simulink model "Drone2_simulink_old1"  (R2024b)
settings: Solver=ode1be  StartTime=0.0  StopTime=1200  FixedStep=0.001  MaxStep=0.001  MinStep=0.00095  RelTol=1e-3
undefined symbols (not defined in the file): DiscIntNeverNeededParam, Environment, Newton, Raphson, Sim3dSensor, Vehicle, X, Y, Z
libraries: sm_lib x2951, nesl_utility x76, slpidlib x25, simulink x4, eeGeneralControl x4, matrix_library x3, rllib x2, sim3dlib x2, uavsim3dlib x2, dspstat3 x1, SignalEditorBlockLib x1, sharedutil x1
(part 10 of 21)

== system Drone2_simulink_old1/Drive Controls/Thrust Controls/Depth and Pitch Control/Main Propellers Thrust Offset Compensation ==
  PPf : Inport
  SPf : Inport  Port=2
  Bow Vertical Thruster Moment Arm : Constant  Value=-Vehicle.Thruster.BVarmX
  Main Propellers Moment Arm : Constant  Value=-Vehicle.Prop.SParmZ
  Product : Product
  Product1 : Product
  Product2 : Product  Inputs=*/
  Stern Vertical Thruster Moment Arm : Constant  Value=Vehicle.Thruster.SVarmX
  Sum : Sum  Inputs=|++
  Sum1 : Sum  Inputs=|++
  VTf : Outport
  wires:
  Product1/1 -> Sum/1
  Product/1 -> Sum/2
  SPf/1 -> Product/1
  PPf/1 -> Product1/1
  Main Propellers Moment Arm/1 -> Product1/2, Product/2
  Bow Vertical Thruster Moment Arm/1 -> Sum1/1
  Stern Vertical Thruster Moment Arm/1 -> Sum1/2
  Sum/1 -> Product2/1
  Sum1/1 -> Product2/2
  Product2/1 -> VTf/1

== system Drone2_simulink_old1/Drive Controls/Thrust Controls/Heading and Yaw Control/psidot ==
  pqr : Inport
  phithetapsi : Inport  Port=2
  Mux1 : Mux  Inputs=[3 3 3]
  psidot : Fcn  Expr=(u[2]*u[4]+u[3]*u[7])/u[8]
  sincos : Trigonometry  Operator=sincos
  psid : Outport  Unit=rad/s  InitialOutput=0  VectorParamsAs1DForOutWhenUnconnected=off
  wires:
  sincos/2 -> Mux1/3
  sincos/1 -> Mux1/2
  phithetapsi/1 -> sincos/1
  pqr/1 -> Mux1/1
  Mux1/1 -> psidot/1
  psidot/1 -> psid/1

== system Drone2_simulink_old1/Drive Controls/Thrust Controls/Heading and Yaw Control/side slip compensation ==
  note: NOTE: Lateral force offset is distributed based of the horizontal thrusters moment arms to make the net torque contribution zero
  v : Inport
  BowHTForce : Gain  Gain=Vehicle.Thruster.SHarmX/(-Vehicle.Thruster.BHarmX+Vehicle.Thruster.SHarmX)
  Gain1 : Gain  Gain=-1
  PIv : slpidlib/PID Controller  Controller=PI  Form=Parallel  TimeDomain=Continuous-time  UseExternalTs=off  SampleTime=-1  IntegratorMethod=Forward Euler  FilterMethod=Forward Euler  ControllerParametersSource=internal  P=10  I=0.01  UseKiTs=off  D=0  UseExternalDerivativeSource=off  N=100  UseFilter=on  TunerSelectOption=Transfer Function Based (PID Tuner App)  InitialConditionSource=internal  InitialConditionForIntegrator=0  InitialConditionForFilter=0  DifferentiatorICPrevScaledInput=0  ExternalReset=none  TrackingMode=off  Kt=1  LimitOutput=off  SatLimitsSource=internal  UpperSaturationLimit=inf  LowerSaturationLimit=-inf  LinearizeAsGain=on  AntiWindupMode=none  Kb=1  LimitIntegrator=off  UpperIntegratorSaturationLimit=inf  LowerIntegratorSaturationLimit=-inf  POutMin=[]  POutMax=[]  IOutMin=[]  IOutMax=[]  DOutMin=[]  DOutMax=[]  NOutMin=[]  NOutMax=[]  SumOutMin=[]  SumOutMax=[]  SaturationOutMin=[]  SaturationOutMax=[]  PParamMin=[]  PParamMax=[]  IParamMin=[]  IParamMax=[]  DParamMin=[]  DParamMax=[]  NParamMin=[]  NParamMax=[]  KbParamMin=[]  KbParamMax=[]  KtParamMin=[]  KtParamMax=[]  KbOutMin=[]  KbOutMax=[]  KtOutMin=[]  KtOutMax=[]  IntegratorOutMin=[]  IntegratorOutMax=[]  FilterOutMin=[]  FilterOutMax=[]  SumI1OutMin=[]  SumI1OutMax=[]  SumI2OutMin=[]  SumI2OutMax=[]  SumI3OutMin=[]  SumI3OutMax=[]  SumI4OutMin=[]  SumI4OutMax=[]  SumDOutMin=[]  SumDOutMax=[]  DifferentiatorOutMin=[]  DifferentiatorOutMax=[]  FilterDiffOutCoefMin=[]  FilterDiffOutCoefMax=[]  ReciprocalOutMin=[]  ReciprocalOutMax=[]  SumDenOutMin=[]  SumDenOutMax=[]  SumNumOutMin=[]  SumNumOutMax=[]  DivideOutMin=[]  DivideOutMax=[]  UdiffTsProdOutMin=[]  UdiffTsProdOutMax=[]  NTsProdOutMin=[]  NTsProdOutMax=[]  UintegralTsProdOutMin=[]  UintegralTsProdOutMax=[]  UngainTsProdOutMin=[]  UngainTsProdOutMax=[]  ClampingZeroOutDataTypeStr=Inherit: Inherit via back propagation  ClampingZeroOutMin=[]  ClampingZeroOutMax=[]  FilterDenConstantOutDataTypeStr=Inherit: Inherit via back propagation  FilterDenConstantOutMin=[]  FilterDenConstantOutMax=[]  PCopyOutDataTypeStr=Inherit: Inherit via back propagation  PCopyOutMin=[]  PCopyOutMax=[]  NCopyOutDataTypeStr=Inherit: Inherit via back propagation  NCopyOutMin=[]  NCopyOutMax=[]  IntegratorContinuousStateAttributes=''  IntegratorStateMustResolveToSignalObject=off  IntegratorRTWStateStorageClass=Auto  FilterContinuousStateAttributes=''  FilterStateMustResolveToSignalObject=off  FilterRTWStateStorageClass=Auto  ParallelPVariant=InternalParameters  IdealPVariant=Disabled  IVariant=InternalParameters  DVariant=Disabled  IntegratorVariant=Continuous  SatVariant=Disabled  AWVariant=Passthrough  PCopyVariant=Disabled  TRVariant=Disabled  FdbkBlocksVariant=Forward  IdealPFdbkVariant=Disabled  SatFdbkVariant=Disabled  DerivativeFilterVariant=Disabled  NVariant=Disabled  NCopyVariant=Disabled_SignalSpec  FilterICVariant=Disabled  IntegratorICVariant=InternalICs  ExternalResetVariant=Disabled  TRSumVariant=Passthrough  SumFdbkVariant=Disabled  SumVariant=Sum_PI  TsampFilterVariant=InternalTs  TsampNgainVariant=Passthrough  TsampIntegralVariant=Disabled_SignalSpec  ExternalSaturationOutDataTypeStr=Inherit: Same as second input  DerivativeSourceVariant=Disabled
  SternHTForce : Gain  Gain=-Vehicle.Thruster.BHarmX/(-Vehicle.Thruster.BHarmX+Vehicle.Thruster.SHarmX)
  BHTf : Outport
  SHTf : Outport  Port=2
  wires:
  Gain1/1 -> PIv/1
  SternHTForce/1 -> SHTf/1
  PIv/1 -> BowHTForce/1, SternHTForce/1
  v/1 -> Gain1/1
  BowHTForce/1 -> BHTf/1

== system Drone2_simulink_old1/Hydrostatic & Hydrodynamic Effects/Added Mass Forces/Added Mass/LPfilter ==
  note: NOTE:
      | Using low pass filters with
      | 1 milisecond time constant
      | to break the algebraic loop
  in : Inport
  Demux : Demux  Outputs=6
  LPfilter{1..6} (6 alike) : TransferFcn  Denominator=[0.001 1]
  Mux : Mux  Inputs=6
  out : Outport
  wires:
  Demux/1 -> LPfilter1/1
  Demux/2 -> LPfilter2/1
  in/1 -> Demux/1
  Demux/6 -> LPfilter6/1
  Demux/5 -> LPfilter5/1
  Demux/4 -> LPfilter4/1
  Demux/3 -> LPfilter3/1
  LPfilter1/1 -> Mux/1
  LPfilter2/1 -> Mux/2
  LPfilter3/1 -> Mux/3
  LPfilter4/1 -> Mux/4
  LPfilter5/1 -> Mux/5
  LPfilter6/1 -> Mux/6
  Mux/1 -> out/1

== system Drone2_simulink_old1/Hydrostatic & Hydrodynamic Effects/Added Mass Forces/Coriolis/Ca(V) ==
  note: $a_1 = m_{11}u \\ a_2 = m_{22}v+m_{26}r\\ a_3 = m_{33}w+m_{35}q\\ b_1 = m_{44}p\\ b_2 = m_{53}w+m_{55}q\\ b_3 = m_{62}v+m_{66}r$
  a1 : Inport
  a2 : Inport  Port=2
  a3 : Inport  Port=3
  b1 : Inport  Port=4
  b2 : Inport  Port=5
  b3 : Inport  Port=6
  Matrix Concatenate : Concatenate  NumInputs=6  Mode=Multidimensional array
  row1 : Subsystem
  row2 : Subsystem
  row3 : Subsystem
  row4 : Subsystem
  row5 : Subsystem
  row6 : Subsystem
  Ca(V) : Outport
  wires:
  a2/1 -> row1/1(a2), row3/2(a2), row6/2(a2), row4/1(a2)
  b3/1 -> row5/4(b3), row4/4(b3)
  b2/1 -> row4/3(b2), row6/4(b2)
  a1/1 -> row6/1(a1), row5/1(a1), row3/1(a1), row2/1(a1)
  row1/1(row1) -> Matrix Concatenate/1
  row2/1(row2) -> Matrix Concatenate/2
  row3/1(row3) -> Matrix Concatenate/3
  a3/1 -> row5/2(a3), row4/2(a3), row1/2(a3), row2/2(a3)
  row4/1(row4) -> Matrix Concatenate/4
  b1/1 -> row5/3(b1), row6/3(b1)
  row6/1(row6) -> Matrix Concatenate/6
  row5/1(row5) -> Matrix Concatenate/5
  Matrix Concatenate/1 -> Ca(V)/1

== system Drone2_simulink_old1/Hydrostatic & Hydrodynamic Effects/Drag Sub system/Aerodynamic drag/Area ==
  Area for rotation : Constant  Value=diag([C_x C_y C_z])  mask{C_x=Vehicle.Body.YZArea, C_y=Vehicle.Body.XZArea, C_z=Vehicle.Body.XYArea}
      mask prompts: C_x "Ax"; C_y "Ay"; C_z "Az"
      mask DialogControl DescGroupVar Prompt: Diagonal Matrix
      mask DialogControl DescTextVar Prompt: Provide values of diagonal element tp produce a diagonal matrix
      mask Display: disp('diag([Ax Ay Az])');
  Area for rotation1 : Constant  Value=diag([C_x C_y C_z])  mask{C_x=Vehicle.Body.Hulldiameter/2, C_y=Vehicle.Body.Length/2, C_z=Vehicle.Body.Length/2}
      mask prompts: C_x "Ax"; C_y "Ay"; C_z "Az"
      mask DialogControl DescGroupVar Prompt: Diagonal Matrix
      mask DialogControl DescTextVar Prompt: Provide values of diagonal element tp produce a diagonal matrix
      mask Display: disp('diag([Ax Ay Az])');
  Constant3 : Constant  Value=3
  Power : Math  Operator=pow
  Product2 : Product  Multiplication=Matrix(*)
  Linear : Outport
  Rotational : Outport  Port=2
  wires:
  Area for rotation1/1 -> Power/1
  Constant3/1 -> Power/2
  Area for rotation/1 -> Product2/1, Linear/1
  Power/1 -> Product2/2
  Product2/1 -> Rotational/1

== system Drone2_simulink_old1/Hydrostatic & Hydrodynamic Effects/Drag Sub system/Aerodynamic drag/Subsystem ==
  V_b : Inport
  rho : Inport  Port=2
  Abs : Abs  SaturateOnIntegerOverflow=off
  Product2 : Product
  Product3 : Product
  0.5rhov^2 : Outport
  wires:
  rho/1 -> Product3/2
  V_b/1 -> Abs/1, Product2/1
  Product3/1 -> 0.5rhov^2/1
  Abs/1 -> Product2/2
  Product2/1 -> Product3/1

== system Drone2_simulink_old1/Hydrostatic & Hydrodynamic Effects/Drag Sub system/Aerodynamic drag/Subsystem1 ==
  omega_b : Inport
  rho : Inport  Port=2
  Abs : Abs  SaturateOnIntegerOverflow=off
  Product2 : Product
  Product3 : Product
  0.5rhov^2 : Outport
  wires:
  Abs/1 -> Product2/2
  omega_b/1 -> Product2/1, Abs/1
  Product2/1 -> Product3/1
  rho/1 -> Product3/2
  Product3/1 -> 0.5rhov^2/1

== system Drone2_simulink_old1/Hydrostatic & Hydrodynamic Effects/Drag Sub system/Hydrodyanamic drag/Area ==
  Area for rotation : Constant  Value=diag([C_x C_y C_z])  mask{C_x=Vehicle.Body.YZArea, C_y=Vehicle.Body.XZArea, C_z=Vehicle.Body.XYArea}
      mask prompts: C_x "Ax"; C_y "Ay"; C_z "Az"
      mask DialogControl DescGroupVar Prompt: Diagonal Matrix
      mask DialogControl DescTextVar Prompt: Provide values of diagonal element tp produce a diagonal matrix
      mask Display: disp('diag([Ax Ay Az])');
  Area for rotation1 : Constant  Value=diag([C_x C_y C_z])  mask{C_x=Vehicle.Body.Hulldiameter/2, C_y=Vehicle.Body.Length/2, C_z=Vehicle.Body.Length/2}
      mask prompts: C_x "Ax"; C_y "Ay"; C_z "Az"
      mask DialogControl DescGroupVar Prompt: Diagonal Matrix
      mask DialogControl DescTextVar Prompt: Provide values of diagonal element tp produce a diagonal matrix
      mask Display: disp('diag([Ax Ay Az])');
  Constant3 : Constant  Value=3
  Power : Math  Operator=pow
  Product2 : Product  Multiplication=Matrix(*)
  Linear : Outport
  Rotational : Outport  Port=2
  wires:
  Product2/1 -> Rotational/1
  Area for rotation1/1 -> Power/1
  Constant3/1 -> Power/2
  Area for rotation/1 -> Product2/1, Linear/1
  Power/1 -> Product2/2

== system Drone2_simulink_old1/Hydrostatic & Hydrodynamic Effects/Drag Sub system/Hydrodyanamic drag/Subsystem ==
  V_b : Inport
  rho : Inport  Port=2
  Dot Product : DotProduct  OutDataTypeStr=Inherit: Inherit via internal rule
  Product2 : Product
  Product3 : Product
  Reshape : Reshape  OutputDimensionality=Customize  OutputDimensions=[3,1]
  Sqrt : Sqrt
  Transpose : Math  Operator=transpose
  0.5rhov^2 : Outport
  wires:
  V_b/1 -> Product2/1, Reshape/1, Transpose/1
  Sqrt/1 -> Product2/2
  Transpose/1 -> Dot Product/1
  Dot Product/1 -> Sqrt/1
  Product3/1 -> 0.5rhov^2/1
  Product2/1 -> Product3/1
  rho/1 -> Product3/2
  Reshape/1 -> Dot Product/2

== system Drone2_simulink_old1/Hydrostatic & Hydrodynamic Effects/Drag Sub system/Hydrodyanamic drag/Subsystem1 ==
  omega_b : Inport
  rho : Inport  Port=2
  Dot Product : DotProduct  OutDataTypeStr=Inherit: Inherit via internal rule
  Product2 : Product
  Product3 : Product
  Sqrt : Sqrt
  Transpose : Math  Operator=transpose
  0.5rhov^2 : Outport
  wires:
  rho/1 -> Product3/2
  omega_b/1 -> Transpose/1, Product2/1, Dot Product/1
  Product3/1 -> 0.5rhov^2/1
  Sqrt/1 -> Product2/2
  Product2/1 -> Product3/1
  Dot Product/1 -> Sqrt/1
  Transpose/1 -> Dot Product/2

== system Drone2_simulink_old1/Hydrostatic & Hydrodynamic Effects/Drag Sub system/Subsystem/Subsystem ==
  vector : Inport
  Dot Product : DotProduct  OutDataTypeStr=Inherit: Inherit via internal rule
  Reshape : Reshape  OutputDimensionality=Customize  OutputDimensions=[3,1]
  Sqrt : Sqrt
  Transpose : Math  Operator=transpose
  Magnitude : Outport
  wires:
  Sqrt/1 -> Magnitude/1
  Reshape/1 -> Dot Product/2, Transpose/1
  vector/1 -> Reshape/1
  Transpose/1 -> Dot Product/1
  Dot Product/1 -> Sqrt/1

== system Drone2_simulink_old1/Hydrostatic & Hydrodynamic Effects/Drag Sub system/Subsystem/Subsystem1 ==
  vector : Inport
  Dot Product : DotProduct  OutDataTypeStr=Inherit: Inherit via internal rule
  Reshape : Reshape  OutputDimensionality=Customize  OutputDimensions=[3,1]
  Sqrt : Sqrt
  Transpose : Math  Operator=transpose
  Magnitude : Outport
  wires:
  Dot Product/1 -> Sqrt/1
  Transpose/1 -> Dot Product/1
  vector/1 -> Reshape/1
  Reshape/1 -> Transpose/1, Dot Product/2
  Sqrt/1 -> Magnitude/1

== system Drone2_simulink_old1/Hydrostatic & Hydrodynamic Effects/Drag Sub system/Subsystem/Transition Angular speed ==
  W(z) : Inport
  1mwz : Inport  Port=2
  omegab : Inport  Port=3
  Add : Sum
  Constant : Constant
  Constant1 : Constant  Value=Environment.AirTransitionAgularSpeed
  Constant2 : Constant  Value=Environment.UnderwaterTransitionAngularSpeed
  Exp : Math
  Gain : Gain  Gain=-10/Environment.Transition
  Product : Product
  Product1 : Product
  Reciprocal : Product  Inputs=/
  Subtract : Sum  Inputs=+-
  Subtract2 : Sum
  lambdaomega : Outport
  wires:
  Subtract2/1 -> Reciprocal/1
  Constant/1 -> Subtract2/2
  Exp/1 -> Subtract2/1
  Gain/1 -> Exp/1
  Subtract/1 -> Gain/1
  Reciprocal/1 -> lambdaomega/1
  Add/1 -> Subtract/2
  Constant1/1 -> Product1/2
  1mwz/1 -> Product1/1
  Product/1 -> Add/1
  Constant2/1 -> Product/2
  omegab/1 -> Subtract/1
  W(z)/1 -> Product/1
  Product1/1 -> Add/2

== system Drone2_simulink_old1/Hydrostatic & Hydrodynamic Effects/Drag Sub system/Subsystem/Transition data ==
  Z : Inport
  Constant2 : Constant
  Exp : Math
  Reciprocal : Product  Inputs=/
  Sum : Sum  Inputs=|++
  k : Gain  Gain=10/(Environment.Transition)
  W(z) : Outport
  wires:
  Constant2/1 -> Sum/2
  Reciprocal/1 -> W(z)/1  "W(z)"
  Sum/1 -> Reciprocal/1
  k/1 -> Exp/1
  Z/1 -> k/1
  Exp/1 -> Sum/1

== system Drone2_simulink_old1/Hydrostatic & Hydrodynamic Effects/Drag Sub system/Subsystem/Transition speed ==
  W(z) : Inport
  1mwz : Inport  Port=2
  vb : Inport  Port=3
  Add : Sum
  Constant : Constant
  Constant1 : Constant  Value=Environment.AirTransitionSpeed
  Constant2 : Constant  Value=Environment.UnderwaterTransitionSpeed
  Exp : Math
  Gain : Gain  Gain=-10/Environment.Transition
  Product : Product
  Product1 : Product
  Reciprocal : Product  Inputs=/
  Subtract : Sum  Inputs=+-
  Subtract2 : Sum
  lambdav : Outport
  wires:
  Product1/1 -> Add/2
  W(z)/1 -> Product/1
  vb/1 -> Subtract/1
  Constant2/1 -> Product/2
  Product/1 -> Add/1
  1mwz/1 -> Product1/1
  Constant1/1 -> Product1/2
  Add/1 -> Subtract/2
  Reciprocal/1 -> lambdav/1
  Subtract/1 -> Gain/1
  Gain/1 -> Exp/1
  Exp/1 -> Subtract2/1
  Constant/1 -> Subtract2/2
  Subtract2/1 -> Reciprocal/1

== system Drone2_simulink_old1/Vehicle_Dynamics/COM_Data/Derived Measurements/Body Acceleration ==
  note: Body acceleration resolved on the rotating body frame
      | $A_{bb}= A_{be} + V_b\times{\omega}_b$
  wb : Inport
  Vb : Inport  Port=2
  Abe : Inport  Port=3
  Demux : Demux  Outputs=3
  Sum : Sum  Inputs=|++
  Vb x wb : sharedutil/3x3 Cross Product  aMode=aMode
  Bus Element Out : Outport  PortName=Abb  Element=Abbx
  Bus Element Out1 : Outport  PortName=Abb  Element=Abby
  Bus Element Out2 : Outport  PortName=Abb  Element=Abbz
  wires:
  Vb/1 -> Vb x wb/1
  Sum/1 -> Demux/1
  Vb x wb/1 -> Sum/1
  wb/1 -> Vb x wb/2
  Abe/1 -> Sum/2
  Demux/1 -> Bus Element Out/1
  Demux/2 -> Bus Element Out1/1
  Demux/3 -> Bus Element Out2/1

== system Drone2_simulink_old1/Vehicle_Dynamics/COM_Data/Derived Measurements/Calculate DCM ==
  R : Inport
  DCMeb --> DCMbe : Math  Operator=transpose  SignedPower=on
  Reshape : Reshape  OutputDimensionality=Customize  OutputDimensions=[3,3]
  DCMbe : Outport
  wires:
  Reshape/1 -> DCMeb --> DCMbe/1
  R/1 -> Reshape/1
  DCMeb --> DCMbe/1 -> DCMbe/1

== system Drone2_simulink_old1/Vehicle_Dynamics/COM_Data/Derived Measurements/Euler Angles ==
  note: NOTE:
      | Euler angles values are calculated assuming a ZYX rotation order and using continuous angular velocity integration from a given initial condition.
  pqr : Inport
  Demux : Demux  Outputs=3
  Integrator : Integrator  WrapState=on
  phidot,thetadot,psidot : Subsystem
  phi : Outport  Unit=rad
  theta : Outport  Port=2  Unit=rad
  psi : Outport  Port=3  Unit=rad
  wires:
  pqr/1 -> phidot,thetadot,psidot/1(pqr)
  Demux/2 -> theta/1
  Demux/3 -> psi/1
  Demux/1 -> phi/1
  Integrator/1 -> phidot,thetadot,psidot/2(phithetapsi), Demux/1
  phidot,thetadot,psidot/1(phid thetad psid) -> Integrator/1

== system Drone2_simulink_old1/Vehicle_Dynamics/COM_Data/Derived Measurements/Incidence Angles ==
  Vb : Inport
  "Incidence, Sideslip & Speed" : Subsystem
      mask Display:
      | port_label('input',1,'V_b','texmode','on');
      | port_label('output',1,'\alpha','texmode','on');
      | port_label('output',2,'\beta','texmode','on');
      | port_label('output',3,'V','texmode','on');
  alpha : Outport  Unit=rad
  beta : Outport  Port=2  Unit=rad
  V : Outport  Port=3  Unit=m/s
  wires:
  Vb/1 -> "Incidence, Sideslip & Speed"/1(Vb)
  "Incidence, Sideslip & Speed"/1(Alpha) -> alpha/1
  "Incidence, Sideslip & Speed"/3(V) -> V/1
  "Incidence, Sideslip & Speed"/2(Beta) -> beta/1

== system Drone2_simulink_old1/Vehicle_Dynamics/Drone_Assembly/Arm Assembly/ArmMotor ==
  ARM 1 : Subsystem  mask{X=0.088, Y=0.044, Z=0.06125, Angle=180, x1=0.008, y1=0.005, z1=0.01, x2=0.038, y2=0.005, z2=0.01, x3=0.008, y3=0.025, z3=0.01, x4=0.038, y4=0.025, z4=0.01}
      mask prompts: Angle "Angle in degree"
      mask DialogControl DescTextVar Prompt: provide all data in SI unit and corrinate of  arm with respect to plate and bolts with respect to arm
      mask DialogControl Container4 Prompt: Arm plate
      mask DialogControl Control2 Prompt: Provide all data in SI Unit with respect from Arm plate origin.
      mask DialogControl Bolt1 Prompt: Bolt 1
      mask DialogControl Bolt2 Prompt: Bolt 2
      mask DialogControl Bolt3 Prompt: Bolt 3
      mask DialogControl Bolt4 Prompt: Bolt 4
  ARM 2 : Subsystem  mask{X=0.428, Y=0.044, Z=0.06125, Angle=180, x1=0.008, y1=0.005, z1=0.01, x2=0.038, y2=0.005, z2=0.01, x3=0.008, y3=0.025, z3=0.01, x4=0.038, y4=0.025, z4=0.01}
      mask prompts: Angle "Angle in degree"
      mask DialogControl DescTextVar Prompt: provide all data in SI unit and corrinate of  arm with respect to plate and bolts with respect to arm
      mask DialogControl Container4 Prompt: Arm plate
      mask DialogControl Control2 Prompt: Provide all data in SI Unit with respect from Arm plate origin.
      mask DialogControl Bolt1 Prompt: Bolt 1
      mask DialogControl Bolt2 Prompt: Bolt 2
      mask DialogControl Bolt3 Prompt: Bolt 3
      mask DialogControl Bolt4 Prompt: Bolt 4
  ARM 3 : Subsystem  mask{X=0.372, Y=0.156, Z=0.06125, Angle=0, x1=0.008, y1=0.005, z1=0.01, x2=0.038, y2=0.005, z2=0.01, x3=0.008, y3=0.025, z3=0.01, x4=0.038, y4=0.025, z4=0.01}
      mask prompts: Angle "Angle in degree"
      mask DialogControl DescTextVar Prompt: provide all data in SI unit and corrinate of  arm with respect to plate and bolts with respect to arm
      mask DialogControl Container4 Prompt: Arm plate
      mask DialogControl Control2 Prompt: Provide all data in SI Unit with respect from Arm plate origin.
      mask DialogControl Bolt1 Prompt: Bolt 1
      mask DialogControl Bolt2 Prompt: Bolt 2
      mask DialogControl Bolt3 Prompt: Bolt 3
      mask DialogControl Bolt4 Prompt: Bolt 4
  ARM 4 : Subsystem  mask{X=0.032, Y=0.156, Z=0.06125, Angle=0, x1=0.008, y1=0.005, z1=0.01, x2=0.038, y2=0.005, z2=0.01, x3=0.008, y3=0.025, z3=0.01, x4=0.038, y4=0.025, z4=0.01}
      mask prompts: Angle "Angle in degree"
      mask DialogControl DescTextVar Prompt: provide all data in SI unit and corrinate of  arm with respect to plate and bolts with respect to arm
      mask DialogControl Container4 Prompt: Arm plate
      mask DialogControl Control2 Prompt: Provide all data in SI Unit with respect from Arm plate origin.
      mask DialogControl Bolt1 Prompt: Bolt 1
      mask DialogControl Bolt2 Prompt: Bolt 2
      mask DialogControl Bolt3 Prompt: Bolt 3
      mask DialogControl Bolt4 Prompt: Bolt 4
  ArmtoMotor{1..4} (4 alike) : sm_lib/Frames and Transforms/Rigid Transform  RotationMethod=None  FollAlignAxisA=+X  BaseAlignAxisA=+Y  FollAlignAxisB=+Y  BaseAlignAxisB=+Z  RotationStandardAxis=+Z  RotationAngle=0  RotationAngleUnits=deg  RotationArbitraryAxis=[0 0 1]  RotationSequenceAxes=FollowerAxes  RotationSequence=XYX  RotationSequenceAngles=[0 0 0]  RotationSequenceAnglesUnits=deg  RotationMatrix=[1 0 0;0 1 0;0 0 1]  Quaternion=[1 0 0 0]  TranslationMethod=Cartesian  TranslationCartesianOffset=[-0.0275 -0.0275 0]  TranslationCartesianOffsetUnits=m  TranslationStandardAxis=+Z  TranslationStandardOffset=0  TranslationStandardOffsetUnits=m  TranslationROffset=0  TranslationROffsetUnits=m  TranslationThetaOffset=0  TranslationThetaOffsetUnits=deg  TranslationZOffset=0  TranslationZOffsetUnits=m
  Motor{1..4} (4 alike) : sm_lib/Body Elements/File Solid  ExtGeomFileName=Motor.STL  UnitType=Custom  ExtGeomFileUnits=mm  StepReaderType=HEX  ExportConvexHullGeometry=off  InertiaType=CalculateFromGeometry  BasedOnType=Density  Density=1780  DensityUnits=kg/m^3  Mass=1  MassUnits=kg  CenterOfMass=[0 0 0]  CenterOfMassUnits=m  MomentsOfInertia=[1 1 1]  MomentsOfInertiaUnits=kg*m^2  ProductsOfInertia=[0 0 0]  ProductsOfInertiaUnits=kg*m^2  GraphicType=FromGeometry  MarkerShape=Sphere  MarkerSize=10  GraphicVisPropType=SimpleVisualProperties  GraphicDiffuseColor=[1.0 0.0 0.2]  GraphicOpacity=1  GraphicSpecularColor=[0.5 0.5 0.5 1.0]  GraphicAmbientColor=[0.15 0.15 0.15 1.0]  GraphicEmissiveColor=[0.0 0.0 0.0 1.0]  GraphicShininess=75  DoExposeReferenceFrame=on  SerializedFrames=<Frames/>
  motortoProp{1..4} (4 alike) : sm_lib/Frames and Transforms/Rigid Transform  RotationMethod=None  FollAlignAxisA=+X  BaseAlignAxisA=+Y  FollAlignAxisB=+Y  BaseAlignAxisB=+Z  RotationStandardAxis=+Z  RotationAngle=0  RotationAngleUnits=deg  RotationArbitraryAxis=[0 0 1]  RotationSequenceAxes=FollowerAxes  RotationSequence=XYX  RotationSequenceAngles=[0 0 0]  RotationSequenceAnglesUnits=deg  RotationMatrix=[1 0 0;0 1 0;0 0 1]  Quaternion=[1 0 0 0]  TranslationMethod=Cartesian  TranslationCartesianOffset=[0 0 0.035]  TranslationCartesianOffsetUnits=m  TranslationStandardAxis=+Z  TranslationStandardOffset=0  TranslationStandardOffsetUnits=m  TranslationROffset=0  TranslationROffsetUnits=m  TranslationThetaOffset=0  TranslationThetaOffsetUnits=deg  TranslationZOffset=0  TranslationZOffsetUnits=m
  Prop1 : PMIOPort  Side=Left
  Prop2 : PMIOPort  Port=2  Side=Left
  Prop4 : PMIOPort  Port=3  Side=Right
  Prop3 : PMIOPort  Port=4  Side=Right
  fromTopPlate : PMIOPort  Port=5  Side=Right
  connections:
  ARM 1/LConn1 -- ARM 2/LConn1 -- ARM 3/LConn1 -- ARM 4/LConn1 -- fromTopPlate/RConn1
  ArmtoMotor1/RConn1 -- Motor1/RConn1
  ArmtoMotor1/LConn1 -- motortoProp1/LConn1 -- ARM 1/RConn1
  ArmtoMotor4/LConn1 -- motortoProp4/LConn1 -- ARM 4/RConn1
  ArmtoMotor4/RConn1 -- Motor4/RConn1
  ArmtoMotor2/LConn1 -- motortoProp2/LConn1 -- ARM 2/RConn1
  ArmtoMotor2/RConn1 -- Motor2/RConn1
  ArmtoMotor3/RConn1 -- Motor3/RConn1
  ArmtoMotor3/LConn1 -- motortoProp3/LConn1 -- ARM 3/RConn1
  Prop1/RConn1 -- motortoProp1/RConn1
  Prop2/RConn1 -- motortoProp2/RConn1
  Prop3/RConn1 -- motortoProp3/RConn1
  Prop4/RConn1 -- motortoProp4/RConn1

== system Drone2_simulink_old1/Vehicle_Dynamics/Drone_Assembly/Arm Assembly/ForceTorqueP1 ==
  Bus Element In : Inport  PortName=MotorRB  Element=Thrust
  Bus Element In1 : Inport  PortName=MotorRB  Element=Torque
  External Force and Torque : sm_lib/Forces and Torques/External Force and Torque  EnableForceX=off  EnableForceY=off  EnableForceZ=on  EnableForce=off  ForceResolutionFrame=AttachedFrame  EnableTorqueX=off  EnableTorqueY=off  EnableTorqueZ=off  EnableTorque=off  TorqueResolutionFrame=AttachedFrame
  Gain : Gain  Gain=Gain
  Revolute Joint : sm_lib/Joints/Revolute Joint  JointMode=Normal  CompositeWrenchDir=FollowerOnBase  CompositeWrenchFrame=BaseFrame  SenseConstraintForce=off  SenseConstraintTorque=off  SenseTotalForce=off  SenseTotalTorque=off  PositionTargetSpecify=off  PositionTargetPriority=High  PositionTargetValue=0  PositionTargetValueUnits=deg  VelocityTargetSpecify=off  VelocityTargetPriority=High  VelocityTargetValue=0  VelocityTargetValueUnits=deg/s  EquilibriumPosition=0  EquilibriumPositionUnits=deg  SpringStiffness=Vehicle.Motor.Stiffness  SpringStiffnessUnits=N*m/deg  DampingCoefficient=Vehicle.Motor.Damping  DampingCoefficientUnits=N*m/(deg/s)  LowerLimitSpecify=off  LowerLimitBound=-90  LowerLimitBoundUnits=deg  LowerLimitStiffness=1e4  LowerLimitStiffnessUnits=N*m/deg  LowerLimitDamping=10  LowerLimitDampingUnits=N*m/(deg/s)  LowerLimitTransitionRegionWidth=0.1  LowerLimitTransitionRegionWidthUnits=deg  UpperLimitSpecify=off  UpperLimitBound=90  UpperLimitBoundUnits=deg  UpperLimitStiffness=1e4  UpperLimitStiffnessUnits=N*m/deg  UpperLimitDamping=10  UpperLimitDampingUnits=N*m/(deg/s)  UpperLimitTransitionRegionWidth=0.1  UpperLimitTransitionRegionWidthUnits=deg  TorqueActuationMode=InputTorque  MotionActuationMode=ComputedMotion  SensePosition=off  SenseVelocity=off  SenseAcceleration=off  SenseTorqueForce=off  SenseLowerLimitTorqueForce=off  SenseUpperLimitTorqueForce=off
  Saturation : Saturate  UpperLimit=Max_Thrust  LowerLimit=Min_Thrust
  Saturation1 : Saturate  UpperLimit=Max_torque  LowerLimit=Min_torque
  Simulink-PS Converter : nesl_utility/Simulink-PS Converter  PhysicalDomain=network_engine_domain  SubClassName=ps_input  LeftPortType=input  RightPortType=output  PseudoPeriodic=off  Frequencies=[]  NoiseDistribution=none  NoiseParameters=[]  Unit=N  AffineConversion=off  FilteringAndDerivatives=provide  SimscapeFilterOrder=1  InputFilterTimeConstant=0.001  UdotUserProvided=0
  Simulink-PS Converter1 : nesl_utility/Simulink-PS Converter  PhysicalDomain=network_engine_domain  SubClassName=ps_input  LeftPortType=input  RightPortType=output  PseudoPeriodic=off  Frequencies=[]  NoiseDistribution=none  NoiseParameters=[]  Unit=N*m  AffineConversion=off  FilteringAndDerivatives=provide  SimscapeFilterOrder=1  InputFilterTimeConstant=0.001  UdotUserProvided=0
  Prop : PMIOPort  Side=Left
  Frommotor : PMIOPort  Port=2  Side=Right
  wires:
  Saturation/1 -> Simulink-PS Converter/1
  Bus Element In/1 -> Saturation/1
  Gain/1 -> Simulink-PS Converter1/1
  Saturation1/1 -> Gain/1
  Bus Element In1/1 -> Saturation1/1
  connections:
  External Force and Torque/RConn1 -- Revolute Joint/LConn1 -- Frommotor/RConn1
  Revolute Joint/LConn2 -- Simulink-PS Converter1/RConn1
  Simulink-PS Converter/RConn1 -- External Force and Torque/LConn1
  Prop/RConn1 -- Revolute Joint/RConn1

== system Drone2_simulink_old1/Vehicle_Dynamics/Drone_Assembly/Arm Assembly/ForceTorqueP2 ==
  Bus Element In : Inport  PortName=MotorRF  Element=Thrust
  Bus Element In1 : Inport  PortName=MotorRF  Element=Torque
  External Force and Torque : sm_lib/Forces and Torques/External Force and Torque  EnableForceX=off  EnableForceY=off  EnableForceZ=on  EnableForce=off  ForceResolutionFrame=AttachedFrame  EnableTorqueX=off  EnableTorqueY=off  EnableTorqueZ=off  EnableTorque=off  TorqueResolutionFrame=AttachedFrame
  Gain : Gain  Gain=Gain
  Revolute Joint : sm_lib/Joints/Revolute Joint  JointMode=Normal  CompositeWrenchDir=FollowerOnBase  CompositeWrenchFrame=BaseFrame  SenseConstraintForce=off  SenseConstraintTorque=off  SenseTotalForce=off  SenseTotalTorque=off  PositionTargetSpecify=off  PositionTargetPriority=High  PositionTargetValue=0  PositionTargetValueUnits=deg  VelocityTargetSpecify=off  VelocityTargetPriority=High  VelocityTargetValue=0  VelocityTargetValueUnits=deg/s  EquilibriumPosition=0  EquilibriumPositionUnits=deg  SpringStiffness=Vehicle.Motor.Stiffness  SpringStiffnessUnits=N*m/deg  DampingCoefficient=Vehicle.Motor.Damping  DampingCoefficientUnits=N*m/(deg/s)  LowerLimitSpecify=off  LowerLimitBound=-90  LowerLimitBoundUnits=deg  LowerLimitStiffness=1e4  LowerLimitStiffnessUnits=N*m/deg  LowerLimitDamping=10  LowerLimitDampingUnits=N*m/(deg/s)  LowerLimitTransitionRegionWidth=0.1  LowerLimitTransitionRegionWidthUnits=deg  UpperLimitSpecify=off  UpperLimitBound=90  UpperLimitBoundUnits=deg  UpperLimitStiffness=1e4  UpperLimitStiffnessUnits=N*m/deg  UpperLimitDamping=10  UpperLimitDampingUnits=N*m/(deg/s)  UpperLimitTransitionRegionWidth=0.1  UpperLimitTransitionRegionWidthUnits=deg  TorqueActuationMode=InputTorque  MotionActuationMode=ComputedMotion  SensePosition=off  SenseVelocity=off  SenseAcceleration=off  SenseTorqueForce=off  SenseLowerLimitTorqueForce=off  SenseUpperLimitTorqueForce=off
  Saturation : Saturate  UpperLimit=Max_Thrust  LowerLimit=Min_Thrust
  Saturation1 : Saturate  UpperLimit=Max_torque  LowerLimit=Min_torque
  Simulink-PS Converter : nesl_utility/Simulink-PS Converter  PhysicalDomain=network_engine_domain  SubClassName=ps_input  LeftPortType=input  RightPortType=output  PseudoPeriodic=off  Frequencies=[]  NoiseDistribution=none  NoiseParameters=[]  Unit=N  AffineConversion=off  FilteringAndDerivatives=provide  SimscapeFilterOrder=1  InputFilterTimeConstant=0.001  UdotUserProvided=0
  Simulink-PS Converter1 : nesl_utility/Simulink-PS Converter  PhysicalDomain=network_engine_domain  SubClassName=ps_input  LeftPortType=input  RightPortType=output  PseudoPeriodic=off  Frequencies=[]  NoiseDistribution=none  NoiseParameters=[]  Unit=N*m  AffineConversion=off  FilteringAndDerivatives=provide  SimscapeFilterOrder=1  InputFilterTimeConstant=0.001  UdotUserProvided=0
  Prop : PMIOPort  Side=Left
  Frommotor : PMIOPort  Port=2  Side=Right
  wires:
  Bus Element In1/1 -> Saturation1/1
  Saturation1/1 -> Gain/1
  Gain/1 -> Simulink-PS Converter1/1
  Bus Element In/1 -> Saturation/1
  Saturation/1 -> Simulink-PS Converter/1
  connections:
  Prop/RConn1 -- Revolute Joint/RConn1
  Simulink-PS Converter/RConn1 -- External Force and Torque/LConn1
  Revolute Joint/LConn2 -- Simulink-PS Converter1/RConn1
  Revolute Joint/LConn1 -- Frommotor/RConn1 -- External Force and Torque/RConn1

== system Drone2_simulink_old1/Vehicle_Dynamics/Drone_Assembly/Arm Assembly/ForceTorqueP3 ==
  Bus Element In : Inport  PortName=MotorLF  Element=Thrust
  Bus Element In1 : Inport  PortName=MotorLF  Element=Torque
  External Force and Torque : sm_lib/Forces and Torques/External Force and Torque  EnableForceX=off  EnableForceY=off  EnableForceZ=on  EnableForce=off  ForceResolutionFrame=AttachedFrame  EnableTorqueX=off  EnableTorqueY=off  EnableTorqueZ=off  EnableTorque=off  TorqueResolutionFrame=AttachedFrame
  Gain : Gain  Gain=Gain
  Revolute Joint : sm_lib/Joints/Revolute Joint  JointMode=Normal  CompositeWrenchDir=FollowerOnBase  CompositeWrenchFrame=BaseFrame  SenseConstraintForce=off  SenseConstraintTorque=off  SenseTotalForce=off  SenseTotalTorque=off  PositionTargetSpecify=off  PositionTargetPriority=High  PositionTargetValue=0  PositionTargetValueUnits=deg  VelocityTargetSpecify=off  VelocityTargetPriority=High  VelocityTargetValue=0  VelocityTargetValueUnits=deg/s  EquilibriumPosition=0  EquilibriumPositionUnits=deg  SpringStiffness=Vehicle.Motor.Stiffness  SpringStiffnessUnits=N*m/deg  DampingCoefficient=Vehicle.Motor.Damping  DampingCoefficientUnits=N*m/(deg/s)  LowerLimitSpecify=off  LowerLimitBound=-90  LowerLimitBoundUnits=deg  LowerLimitStiffness=1e4  LowerLimitStiffnessUnits=N*m/deg  LowerLimitDamping=10  LowerLimitDampingUnits=N*m/(deg/s)  LowerLimitTransitionRegionWidth=0.1  LowerLimitTransitionRegionWidthUnits=deg  UpperLimitSpecify=off  UpperLimitBound=90  UpperLimitBoundUnits=deg  UpperLimitStiffness=1e4  UpperLimitStiffnessUnits=N*m/deg  UpperLimitDamping=10  UpperLimitDampingUnits=N*m/(deg/s)  UpperLimitTransitionRegionWidth=0.1  UpperLimitTransitionRegionWidthUnits=deg  TorqueActuationMode=InputTorque  MotionActuationMode=ComputedMotion  SensePosition=off  SenseVelocity=off  SenseAcceleration=off  SenseTorqueForce=off  SenseLowerLimitTorqueForce=off  SenseUpperLimitTorqueForce=off
  Saturation : Saturate  UpperLimit=Max_Thrust  LowerLimit=Min_Thrust
  Saturation1 : Saturate  UpperLimit=Max_torque  LowerLimit=Min_torque
  Simulink-PS Converter : nesl_utility/Simulink-PS Converter  PhysicalDomain=network_engine_domain  SubClassName=ps_input  LeftPortType=input  RightPortType=output  PseudoPeriodic=off  Frequencies=[]  NoiseDistribution=none  NoiseParameters=[]  Unit=N  AffineConversion=off  FilteringAndDerivatives=provide  SimscapeFilterOrder=1  InputFilterTimeConstant=0.001  UdotUserProvided=0
  Simulink-PS Converter1 : nesl_utility/Simulink-PS Converter  PhysicalDomain=network_engine_domain  SubClassName=ps_input  LeftPortType=input  RightPortType=output  PseudoPeriodic=off  Frequencies=[]  NoiseDistribution=none  NoiseParameters=[]  Unit=N*m  AffineConversion=off  FilteringAndDerivatives=provide  SimscapeFilterOrder=1  InputFilterTimeConstant=0.001  UdotUserProvided=0
  Prop : PMIOPort  Side=Left
  Frommotor : PMIOPort  Port=2  Side=Right
  wires:
  Saturation/1 -> Simulink-PS Converter/1
  Bus Element In/1 -> Saturation/1
  Gain/1 -> Simulink-PS Converter1/1
  Saturation1/1 -> Gain/1
  Bus Element In1/1 -> Saturation1/1
  connections:
  External Force and Torque/RConn1 -- Frommotor/RConn1 -- Revolute Joint/LConn1
  Revolute Joint/LConn2 -- Simulink-PS Converter1/RConn1
  Simulink-PS Converter/RConn1 -- External Force and Torque/LConn1
  Prop/RConn1 -- Revolute Joint/RConn1

== system Drone2_simulink_old1/Vehicle_Dynamics/Drone_Assembly/Arm Assembly/ForceTorqueP4 ==
  Bus Element In : Inport  PortName=MotorLB  Element=Thrust
  Bus Element In1 : Inport  PortName=MotorLB  Element=Torque
  External Force and Torque : sm_lib/Forces and Torques/External Force and Torque  EnableForceX=off  EnableForceY=off  EnableForceZ=on  EnableForce=off  ForceResolutionFrame=AttachedFrame  EnableTorqueX=off  EnableTorqueY=off  EnableTorqueZ=off  EnableTorque=off  TorqueResolutionFrame=AttachedFrame
  Gain : Gain  Gain=Gain
  Revolute Joint : sm_lib/Joints/Revolute Joint  JointMode=Normal  CompositeWrenchDir=FollowerOnBase  CompositeWrenchFrame=BaseFrame  SenseConstraintForce=off  SenseConstraintTorque=off  SenseTotalForce=off  SenseTotalTorque=off  PositionTargetSpecify=off  PositionTargetPriority=High  PositionTargetValue=0  PositionTargetValueUnits=deg  VelocityTargetSpecify=off  VelocityTargetPriority=High  VelocityTargetValue=0  VelocityTargetValueUnits=deg/s  EquilibriumPosition=0  EquilibriumPositionUnits=deg  SpringStiffness=Vehicle.Motor.Stiffness  SpringStiffnessUnits=N*m/deg  DampingCoefficient=Vehicle.Motor.Damping  DampingCoefficientUnits=N*m/(deg/s)  LowerLimitSpecify=off  LowerLimitBound=-90  LowerLimitBoundUnits=deg  LowerLimitStiffness=1e4  LowerLimitStiffnessUnits=N*m/deg  LowerLimitDamping=10  LowerLimitDampingUnits=N*m/(deg/s)  LowerLimitTransitionRegionWidth=0.1  LowerLimitTransitionRegionWidthUnits=deg  UpperLimitSpecify=off  UpperLimitBound=90  UpperLimitBoundUnits=deg  UpperLimitStiffness=1e4  UpperLimitStiffnessUnits=N*m/deg  UpperLimitDamping=10  UpperLimitDampingUnits=N*m/(deg/s)  UpperLimitTransitionRegionWidth=0.1  UpperLimitTransitionRegionWidthUnits=deg  TorqueActuationMode=InputTorque  MotionActuationMode=ComputedMotion  SensePosition=off  SenseVelocity=off  SenseAcceleration=off  SenseTorqueForce=off  SenseLowerLimitTorqueForce=off  SenseUpperLimitTorqueForce=off
  Saturation : Saturate  UpperLimit=Max_Thrust  LowerLimit=Min_Thrust
  Saturation1 : Saturate  UpperLimit=Max_torque  LowerLimit=Min_torque
  Simulink-PS Converter : nesl_utility/Simulink-PS Converter  PhysicalDomain=network_engine_domain  SubClassName=ps_input  LeftPortType=input  RightPortType=output  PseudoPeriodic=off  Frequencies=[]  NoiseDistribution=none  NoiseParameters=[]  Unit=N  AffineConversion=off  FilteringAndDerivatives=provide  SimscapeFilterOrder=1  InputFilterTimeConstant=0.001  UdotUserProvided=0
  Simulink-PS Converter1 : nesl_utility/Simulink-PS Converter  PhysicalDomain=network_engine_domain  SubClassName=ps_input  LeftPortType=input  RightPortType=output  PseudoPeriodic=off  Frequencies=[]  NoiseDistribution=none  NoiseParameters=[]  Unit=N*m  AffineConversion=off  FilteringAndDerivatives=provide  SimscapeFilterOrder=1  InputFilterTimeConstant=0.001  UdotUserProvided=0
  Prop : PMIOPort  Side=Left
  Frommotor : PMIOPort  Port=2  Side=Right
  wires:
  Bus Element In1/1 -> Saturation1/1
  Saturation1/1 -> Gain/1
  Gain/1 -> Simulink-PS Converter1/1
  Bus Element In/1 -> Saturation/1
  Saturation/1 -> Simulink-PS Converter/1
  connections:
  Prop/RConn1 -- Revolute Joint/RConn1
  Simulink-PS Converter/RConn1 -- External Force and Torque/LConn1
  Revolute Joint/LConn2 -- Simulink-PS Converter1/RConn1
  Revolute Joint/LConn1 -- Frommotor/RConn1 -- External Force and Torque/RConn1

== system Drone2_simulink_old1/Vehicle_Dynamics/Drone_Assembly/Arm Assembly/Landing gear ==
  Landing Gear1 : Subsystem  mask{Xtl=0.025, Ytl=-0.006, Ztl=-0.15125, X=0.025, Y=0.025, Z=0.0985, x_dist=0.03, y_dist=0.02}
      mask prompts: Xtl "X cord"; Ytl "Y cord"; Ztl "Z cord"; X "X cord"; Y "Y cord"; Z "Z cord"; x_dist "X dist"; y_dist "Y dist"
      mask DialogControl Container4 Prompt: top plate to landing gear
      mask DialogControl Container5 Prompt: Landing gear to first hole
      mask DialogControl Container6 Prompt: Hole patern
  Landing Gear2 : Subsystem  mask{Xtl=0.365, Ytl=-0.006, Ztl=-0.15125, X=0.025, Y=0.025, Z=0.0985, x_dist=0.03, y_dist=0.02}
      mask prompts: Xtl "X cord"; Ytl "Y cord"; Ztl "Z cord"; X "X cord"; Y "Y cord"; Z "Z cord"; x_dist "X dist"; y_dist "Y dist"
      mask DialogControl Container4 Prompt: top plate to landing gear
      mask DialogControl Container5 Prompt: Landing gear to first hole
      mask DialogControl Container6 Prompt: Hole patern
  Landing Gear3 : Subsystem  mask{Xtl=0.025, Ytl=0.146, Ztl=-0.15125, X=0.025, Y=0.025, Z=0.0985, x_dist=0.03, y_dist=0.02}
      mask prompts: Xtl "X cord"; Ytl "Y cord"; Ztl "Z cord"; X "X cord"; Y "Y cord"; Z "Z cord"; x_dist "X dist"; y_dist "Y dist"
      mask DialogControl Container4 Prompt: top plate to landing gear
      mask DialogControl Container5 Prompt: Landing gear to first hole
      mask DialogControl Container6 Prompt: Hole patern
  Landing Gear4 : Subsystem  mask{Xtl=0.365, Ytl=0.146, Ztl=-0.15125, X=0.025, Y=0.025, Z=0.0985, x_dist=0.03, y_dist=0.02}
      mask prompts: Xtl "X cord"; Ytl "Y cord"; Ztl "Z cord"; X "X cord"; Y "Y cord"; Z "Z cord"; x_dist "X dist"; y_dist "Y dist"
      mask DialogControl Container4 Prompt: top plate to landing gear
      mask DialogControl Container5 Prompt: Landing gear to first hole
      mask DialogControl Container6 Prompt: Hole patern
  FromTopPlate : PMIOPort  Side=Right
  connections:
  Landing Gear1/LConn1 -- FromTopPlate/RConn1 -- Landing Gear2/LConn1 -- Landing Gear4/LConn1 -- Landing Gear3/LConn1

== system Drone2_simulink_old1/Vehicle_Dynamics/Drone_Assembly/Arm Assembly/M8Nutbolat on plates ==
  M8 AssemblyR1 : Subsystem  mask{X=0, Y=0, Z=0}
  M8 AssemblyR2 : Subsystem  mask{X=0.1, Y=0, Z=0}
  M8 AssemblyR3 : Subsystem  mask{X=0.325, Y=0, Z=0}
  M8 AssemblyR4 : Subsystem  mask{X=0.425, Y=0, Z=0}
  M8 AssemblyR5 : Subsystem  mask{X=0, Y=0.176, Z=0}
  M8 AssemblyR6 : Subsystem  mask{X=0.1, Y=0.176, Z=0}
  M8 AssemblyR7 : Subsystem  mask{X=0.325, Y=0.176, Z=0}
  M8 AssemblyR8 : Subsystem  mask{X=.425, Y=0.176, Z=0}
  firstholeR1 : PMIOPort  Side=Left
  connections:
  M8 AssemblyR4/LConn1 -- M8 AssemblyR1/LConn1 -- M8 AssemblyR5/LConn1 -- firstholeR1/RConn1 -- M8 AssemblyR2/LConn1 -- M8 AssemblyR6/LConn1 -- M8 AssemblyR3/LConn1 -- M8 AssemblyR7/LConn1 -- M8 AssemblyR8/LConn1

== system Drone2_simulink_old1/Vehicle_Dynamics/Drone_Assembly/Cylinder_Assembly/BackCap ==
  Acap2 : sm_lib/Body Elements/File Solid  ExtGeomFileName=Acrylic_cap.STL  UnitType=Custom  ExtGeomFileUnits=mm  StepReaderType=HEX  ExportConvexHullGeometry=off  InertiaType=CalculateFromGeometry  BasedOnType=Density  Density=1200  DensityUnits=kg/m^3  Mass=1  MassUnits=kg  CenterOfMass=[0 0 0]  CenterOfMassUnits=m  MomentsOfInertia=[1 1 1]  MomentsOfInertiaUnits=kg*m^2  ProductsOfInertia=[0 0 0]  ProductsOfInertiaUnits=kg*m^2  GraphicType=FromGeometry  MarkerShape=Sphere  MarkerSize=10  GraphicVisPropType=SimpleVisualProperties  GraphicDiffuseColor=[0.6 0.4 1.0]  GraphicOpacity=0.5  GraphicSpecularColor=[0.5 0.5 0.5 1.0]  GraphicAmbientColor=[0.15 0.15 0.15 1.0]  GraphicEmissiveColor=[0.0 0.0 0.0 1.0]  GraphicShininess=75  DoExposeReferenceFrame=on  SerializedFrames=<Frames/>
  Centre to OringW21 : sm_lib/Frames and Transforms/Rigid Transform  RotationMethod=None  FollAlignAxisA=+X  BaseAlignAxisA=+Y  FollAlignAxisB=+Y  BaseAlignAxisB=+Z  RotationStandardAxis=+Z  RotationAngle=180  RotationAngleUnits=deg  RotationArbitraryAxis=[0 0 1]  RotationSequenceAxes=FollowerAxes  RotationSequence=XYX  RotationSequenceAngles=[0 0 0]  RotationSequenceAnglesUnits=deg  RotationMatrix=[1 0 0;0 1 0;0 0 1]  Quaternion=[1 0 0 0]  TranslationMethod=Cartesian  TranslationCartesianOffset=[-0.216 -0.075485 -0.075485]  TranslationCartesianOffsetUnits=m  TranslationStandardAxis=+Z  TranslationStandardOffset=0  TranslationStandardOffsetUnits=m  TranslationROffset=0  TranslationROffsetUnits=m  TranslationThetaOffset=0  TranslationThetaOffsetUnits=deg  TranslationZOffset=0  TranslationZOffsetUnits=m
  Centre to WoodcapF : sm_lib/Frames and Transforms/Rigid Transform  RotationMethod=None  FollAlignAxisA=+X  BaseAlignAxisA=+Y  FollAlignAxisB=+Y  BaseAlignAxisB=+Z  RotationStandardAxis=+Z  RotationAngle=180  RotationAngleUnits=deg  RotationArbitraryAxis=[0 0 1]  RotationSequenceAxes=FollowerAxes  RotationSequence=XYX  RotationSequenceAngles=[0 0 0]  RotationSequenceAnglesUnits=deg  RotationMatrix=[1 0 0;0 1 0;0 0 1]  Quaternion=[1 0 0 0]  TranslationMethod=Cartesian  TranslationCartesianOffset=[-0.223 -0.0747394 -0.0745]  TranslationCartesianOffsetUnits=m  TranslationStandardAxis=+Z  TranslationStandardOffset=0  TranslationStandardOffsetUnits=m  TranslationROffset=0  TranslationROffsetUnits=m  TranslationThetaOffset=0  TranslationThetaOffsetUnits=deg  TranslationZOffset=0  TranslationZOffsetUnits=m
  Centre to washercentre : sm_lib/Frames and Transforms/Rigid Transform  RotationMethod=None  FollAlignAxisA=+X  BaseAlignAxisA=+Y  FollAlignAxisB=+Y  BaseAlignAxisB=+Z  RotationStandardAxis=+Z  RotationAngle=180  RotationAngleUnits=deg  RotationArbitraryAxis=[0 0 1]  RotationSequenceAxes=FollowerAxes  RotationSequence=XYX  RotationSequenceAngles=[0 0 0]  RotationSequenceAnglesUnits=deg  RotationMatrix=[1 0 0;0 1 0;0 0 1]  Quaternion=[1 0 0 0]  TranslationMethod=Cartesian  TranslationCartesianOffset=[-0.227 0 0]  TranslationCartesianOffsetUnits=m  TranslationStandardAxis=+Z  TranslationStandardOffset=0  TranslationStandardOffsetUnits=m  TranslationROffset=0  TranslationROffsetUnits=m  TranslationThetaOffset=0  TranslationThetaOffsetUnits=deg  TranslationZOffset=0  TranslationZOffsetUnits=m
  Centre toOringW22 : sm_lib/Frames and Transforms/Rigid Transform  RotationMethod=None  FollAlignAxisA=+X  BaseAlignAxisA=+Y  FollAlignAxisB=+Y  BaseAlignAxisB=+Z  RotationStandardAxis=+Z  RotationAngle=180  RotationAngleUnits=deg  RotationArbitraryAxis=[0 0 1]  RotationSequenceAxes=FollowerAxes  RotationSequence=XYX  RotationSequenceAngles=[0 0 0]  RotationSequenceAnglesUnits=deg  RotationMatrix=[1 0 0;0 1 0;0 0 1]  Quaternion=[1 0 0 0]  TranslationMethod=Cartesian  TranslationCartesianOffset=[0.008 0 0]  TranslationCartesianOffsetUnits=m  TranslationStandardAxis=+Z  TranslationStandardOffset=0  TranslationStandardOffsetUnits=m  TranslationROffset=0  TranslationROffsetUnits=m  TranslationThetaOffset=0  TranslationThetaOffsetUnits=deg  TranslationZOffset=0  TranslationZOffsetUnits=m
  Nut on Cap : Subsystem
      mask Display: image('socket head cap screw_isM3.PNG');
  Oring_W21 : sm_lib/Body Elements/File Solid  ExtGeomFileName=O-ring.STL  UnitType=Custom  ExtGeomFileUnits=mm  StepReaderType=HEX  ExportConvexHullGeometry=off  InertiaType=CalculateFromGeometry  BasedOnType=Density  Density=1250  DensityUnits=kg/m^3  Mass=1  MassUnits=kg  CenterOfMass=[0 0 0]  CenterOfMassUnits=m  MomentsOfInertia=[1 1 1]  MomentsOfInertiaUnits=kg*m^2  ProductsOfInertia=[0 0 0]  ProductsOfInertiaUnits=kg*m^2  GraphicType=FromGeometry  MarkerShape=Sphere  MarkerSize=10  GraphicVisPropType=SimpleVisualProperties  GraphicDiffuseColor=[0.0 0.0 0.0]  GraphicOpacity=1  GraphicSpecularColor=[0.5 0.5 0.5 1.0]  GraphicAmbientColor=[0.15 0.15 0.15 1.0]  GraphicEmissiveColor=[0.0 0.0 0.0 1.0]  GraphicShininess=75  DoExposeReferenceFrame=on  SerializedFrames=<Frames/>
  Oring_W22 : sm_lib/Body Elements/File Solid  ExtGeomFileName=O-ring.STL  UnitType=Custom  ExtGeomFileUnits=mm  StepReaderType=HEX  ExportConvexHullGeometry=off  InertiaType=CalculateFromGeometry  BasedOnType=Density  Density=1250  DensityUnits=kg/m^3  Mass=1  MassUnits=kg  CenterOfMass=[0 0 0]  CenterOfMassUnits=m  MomentsOfInertia=[1 1 1]  MomentsOfInertiaUnits=kg*m^2  ProductsOfInertia=[0 0 0]  ProductsOfInertiaUnits=kg*m^2  GraphicType=FromGeometry  MarkerShape=Sphere  MarkerSize=10  GraphicVisPropType=SimpleVisualProperties  GraphicDiffuseColor=[0.0 0.0 0.0]  GraphicOpacity=1  GraphicSpecularColor=[0.5 0.5 0.5 1.0]  GraphicAmbientColor=[0.15 0.15 0.15 1.0]  GraphicEmissiveColor=[0.0 0.0 0.0 1.0]  GraphicShininess=75  DoExposeReferenceFrame=on  SerializedFrames=<Frames/>
  Wcap_1 : sm_lib/Body Elements/File Solid  ExtGeomFileName=woden_cap.STL  UnitType=Custom  ExtGeomFileUnits=mm  StepReaderType=HEX  ExportConvexHullGeometry=off  InertiaType=CalculateFromGeometry  BasedOnType=Density  Density=630  DensityUnits=kg/m^3  Mass=1  MassUnits=kg  CenterOfMass=[0 0 0]  CenterOfMassUnits=m  MomentsOfInertia=[1 1 1]  MomentsOfInertiaUnits=kg*m^2  ProductsOfInertia=[0 0 0]  ProductsOfInertiaUnits=kg*m^2  GraphicType=FromGeometry  MarkerShape=Sphere  MarkerSize=10  GraphicVisPropType=SimpleVisualProperties  GraphicDiffuseColor=[0.5019608 0.32156864 0.02745098]  GraphicOpacity=0.5  GraphicSpecularColor=[0.5 0.5 0.5 1.0]  GraphicAmbientColor=[0.15 0.15 0.15 1.0]  GraphicEmissiveColor=[0.0 0.0 0.0 1.0]  GraphicShininess=75  DoExposeReferenceFrame=on  SerializedFrames=<Frames/>
  origintoCap2 : sm_lib/Frames and Transforms/Rigid Transform  RotationMethod=None  FollAlignAxisA=+X  BaseAlignAxisA=+Y  FollAlignAxisB=+Y  BaseAlignAxisB=+Z  RotationStandardAxis=+Z  RotationAngle=0  RotationAngleUnits=deg  RotationArbitraryAxis=[0 0 1]  RotationSequenceAxes=FollowerAxes  RotationSequence=XYX  RotationSequenceAngles=[0 0 0]  RotationSequenceAnglesUnits=deg  RotationMatrix=[1 0 0;0 1 0;0 0 1]  Quaternion=[1 0 0 0]  TranslationMethod=Cartesian  TranslationCartesianOffset=[-0.227 -0.08 -0.0800014]  TranslationCartesianOffsetUnits=m  TranslationStandardAxis=+Z  TranslationStandardOffset=0  TranslationStandardOffsetUnits=m  TranslationROffset=0  TranslationROffsetUnits=m  TranslationThetaOffset=0  TranslationThetaOffsetUnits=deg  TranslationZOffset=0  TranslationZOffsetUnits=m
  washercentre to washer : sm_lib/Frames and Transforms/Rigid Transform  RotationMethod=AlignedAxes  FollAlignAxisA=-X  BaseAlignAxisA=-Z  FollAlignAxisB=+Y  BaseAlignAxisB=+Y  RotationStandardAxis=+Z  RotationAngle=180  RotationAngleUnits=deg  RotationArbitraryAxis=[0 0 1]  RotationSequenceAxes=FollowerAxes  RotationSequence=XYX  RotationSequenceAngles=[0 0 0]  RotationSequenceAnglesUnits=deg  RotationMatrix=[1 0 0;0 1 0;0 0 1]  Quaternion=[1 0 0 0]  TranslationMethod=None  TranslationCartesianOffset=[0.227 0 0]  TranslationCartesianOffsetUnits=m  TranslationStandardAxis=+Z  TranslationStandardOffset=0  TranslationStandardOffsetUnits=m  TranslationROffset=0.675  TranslationROffsetUnits=m  TranslationThetaOffset=0  TranslationThetaOffsetUnits=deg  TranslationZOffset=0.0035  TranslationZOffsetUnits=m
  from_CylinderCentre : PMIOPort  Side=Left
  connections:
  Centre to washercentre/LConn1 -- origintoCap2/LConn1 -- Centre to OringW21/LConn1 -- Centre to WoodcapF/LConn1 -- from_CylinderCentre/RConn1
  Centre toOringW22/RConn1 -- Oring_W22/RConn1
  Centre to washercentre/RConn1 -- washercentre to washer/LConn1
  washercentre to washer/RConn1 -- Nut on Cap/LConn1
  origintoCap2/RConn1 -- Acap2/RConn1
  Centre to OringW21/RConn1 -- Centre toOringW22/LConn1 -- Oring_W21/RConn1
  Centre to WoodcapF/RConn1 -- Wcap_1/RConn1
